simulink model "PID_self1"  (Simulink 8.1)
settings: Solver=ode45  StartTime=0.0  StopTime=0.8  FixedStep=0.000005  MaxStep=5e-4  MinStep=5e-6  RelTol=1e-3
libraries: simulink x2
settings Model: Creator=mainster  LastModifiedBy=mainster

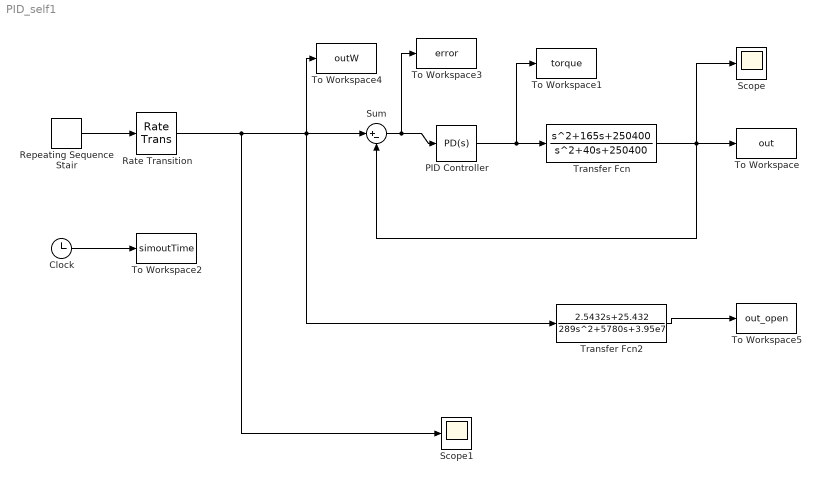
== system PID_self1 ==
  Clock : Clock
  PID Controller : simulink/Continuous/PID Controller  Controller=PD  TimeDomain=Continuous-time  SampleTime=0.0005  IntegratorMethod=Forward Euler  FilterMethod=Forward Euler  Form=Parallel  P=670446.147703758  I=89171.9542391  D=0  N=100  InitialConditionSource=internal  InitialConditionForIntegrator=0  InitialConditionForFilter=1  ExternalReset=none  LimitOutput=off  UpperSaturationLimit=200000  LowerSaturationLimit=-200000  LinearizeAsGain=off  AntiWindupMode=clamping  Kb=1  TrackingMode=on  Kt=1  PParamMin=[]  PParamMax=[]  IParamMin=[]  IParamMax=[]  DParamMin=[]  DParamMax=[]  NParamMin=[]  NParamMax=[]  KbParamMin=[]  KbParamMax=[]  KtParamMin=[]  KtParamMax=[]  POutMin=[]  POutMax=[]  IOutMin=[]  IOutMax=[]  DOutMin=[]  DOutMax=[]  NOutMin=[]  NOutMax=[]  KbOutMin=[]  KbOutMax=[]  KtOutMin=[]  KtOutMax=[]  IntegratorOutMin=[]  IntegratorOutMax=[]  FilterOutMin=[]  FilterOutMax=[]  SumOutMin=[]  SumOutMax=[]  SumI1OutMin=[]  SumI1OutMax=[]  SumI2OutMin=[]  SumI2OutMax=[]  SumI3OutMin=[]  SumI3OutMax=[]  SumDOutMin=[]  SumDOutMax=[]  SaturationOutMin=[]  SaturationOutMax=[]  IntegratorContinuousStateAttributes=''  IntegratorStateMustResolveToSignalObject=off  IntegratorRTWStateStorageClass=Auto  FilterContinuousStateAttributes=''  FilterStateMustResolveToSignalObject=off  FilterRTWStateStorageClass=Auto
  Rate Transition : RateTransition  OutPortSampleTimeMultiple=0.001
  Repeating Sequence Stair : simulink/Sources/Repeating Sequence Stair  OutValues=0.25*[3 -1 6 -2 1 -3 2 1 -6 1].'  tsamp=0.05  OutMin=[]  OutMax=[]  OutDataTypeStr=double  OutputDataTypeScalingMode=double  OutDataType=fixdt(0,8)  ConRadixGroup=Best Precision: Vector-wise  OutScaling=2^-12
  Scope : Scope
  Scope1 : Scope
      settings: TimeRange=0.03000000000000003  YMin=0.25  YMax=0.75
  Sum : Sum  Inputs=|+-
  To Workspace : ToWorkspace  VariableName=out  SampleTime=-1  SaveFormat=Structure
  To Workspace1 : ToWorkspace  VariableName=torque  SampleTime=-1  SaveFormat=Structure
  To Workspace2 : ToWorkspace  VariableName=simoutTime  SampleTime=-1  SaveFormat=Structure
  To Workspace3 : ToWorkspace  VariableName=error  SampleTime=-1  SaveFormat=Structure
  To Workspace4 : ToWorkspace  VariableName=outW  SampleTime=-1  SaveFormat=Structure
  To Workspace5 : ToWorkspace  VariableName=out_open  SampleTime=-1  SaveFormat=Structure
  Transfer Fcn : TransferFcn  Numerator=[1 165 250400]  Denominator=[1 40 250400]
  Transfer Fcn2 : TransferFcn  Numerator=[2.5432 25.432]  Denominator=[289 5780 3.95e7]
  wires:
  PID Controller/1 -> Transfer Fcn/1, To Workspace1/1
  Transfer Fcn/1 -> Sum/2, To Workspace/1, Scope/1
  Sum/1 -> PID Controller/1, To Workspace3/1
  Clock/1 -> To Workspace2/1
  Transfer Fcn2/1 -> To Workspace5/1
  Repeating Sequence Stair/1 -> Rate Transition/1
  Rate Transition/1 -> To Workspace4/1, Sum/1, Transfer Fcn2/1, Scope1/1
